simulink library "lightbar"  (Simulink 8.2)
settings: Solver=ode1  StartTime=0.0  StopTime=Inf  FixedStep=0.001  RelTol=1e-3
PostLoadFcn:
  | , if any(exist('dsrtsu_mdlpostloadfcn', 'file') == [2, 3, 6]), try dsrtsu_mdlpostloadfcn('Execute', bdroot); catch fprintf('Error in PostLoadFcn (dsrtsu_mdlpostloadfcn) for model "%s":\n %s\n', bdroot, lasterr); end, end,
libraries: lightbar x5, simulink x3, srx_platform x2, dsrc_transmitter x1
settings Model: DSRTSU_INTERNAL_RTI_VER=440  DSRTSU_INTERNAL_RTI_TYPE=rti1401  DSRTSU_INTERNAL_RTIFPGA=30  Creator=Admin  LastModifiedBy=Admin

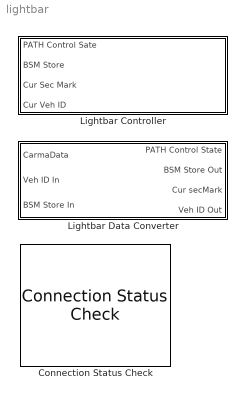
== system lightbar ==
  Connection Status Check : lightbar/Lightbar Controller/Light Control Logic/Connection Check/Connection Status Check
  Lightbar Controller : Subsystem
  Lightbar Data Converter : Subsystem

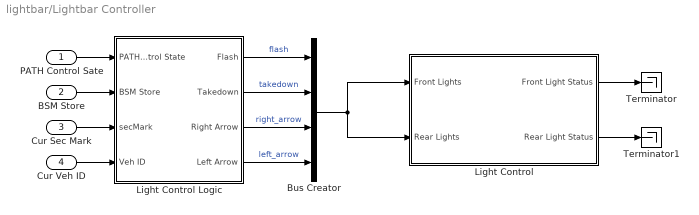
== system lightbar/Lightbar Controller ==
  PATH Control Sate : Inport
  BSM Store : Inport  Port=2
  Cur Sec Mark : Inport  Port=3
  Cur Veh ID : Inport  Port=4
  Bus Creator : BusCreator  Inputs='flash','takedown','right_arrow','left_arrow'  OutDataTypeStr=Bus: LightCommandBus  NonVirtualBus=on
  Light Control : Subsystem
  Light Control Logic : Subsystem
  Terminator : Terminator
  Terminator1 : Terminator
  wires:
  Bus Creator/1 -> Light Control/1(Front Lights), Light Control/2(Rear Lights)
  Light Control Logic/1(Flash) -> Bus Creator/1  "flash"
  Light Control Logic/2(Takedown) -> Bus Creator/2  "takedown"
  Light Control Logic/3(Right Arrow) -> Bus Creator/3  "right_arrow"
  Light Control Logic/4(Left Arrow) -> Bus Creator/4  "left_arrow"
  Light Control/1(Front Light Status) -> Terminator/1
  Light Control/2(Rear Light Status) -> Terminator1/1
  PATH Control Sate/1 -> Light Control Logic/1(PATH Control State)
  BSM Store/1 -> Light Control Logic/2(BSM Store)
  Cur Sec Mark/1 -> Light Control Logic/3(secMark)
  Cur Veh ID/1 -> Light Control Logic/4(Veh ID)

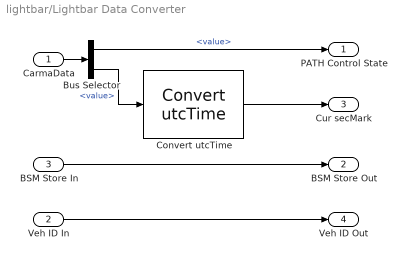
== system lightbar/Lightbar Data Converter ==
  CarmaData : Inport  OutDataTypeStr=Bus: GlobalStoreBus
  Veh ID In : Inport  Port=2
  BSM Store In : Inport  Port=3
  Bus Selector : BusSelector  OutputSignals=path_ctrl_status.value,global_utc_time_s.value
  Convert utcTime : dsrc_transmitter/BSM Broadcast/Convert TORC Data/Data Conversion/Convert utcTime
  PATH Control State : Outport
  BSM Store Out : Outport  Port=2
  Cur secMark : Outport  Port=3
  Veh ID Out : Outport  Port=4
  wires:
  CarmaData/1 -> Bus Selector/1
  Bus Selector/1 -> PATH Control State/1  "<value>"
  Veh ID In/1 -> Veh ID Out/1
  Convert utcTime/1 -> Cur secMark/1
  Bus Selector/2 -> Convert utcTime/1  "<value>"
  BSM Store In/1 -> BSM Store Out/1

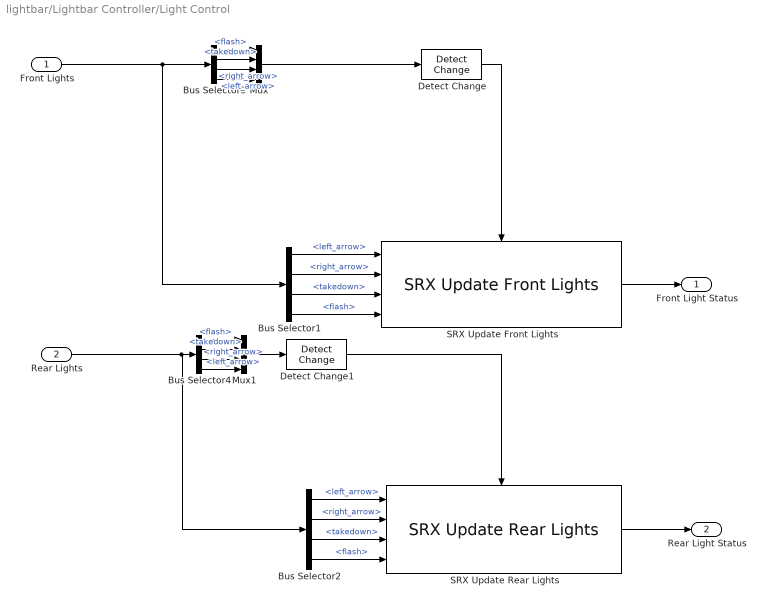
== system lightbar/Lightbar Controller/Light Control ==
  Front Lights : Inport  OutDataTypeStr=Bus: LightCommandBus
  Rear Lights : Inport  Port=2  OutDataTypeStr=Bus: LightCommandBus
  Bus Selector1 : BusSelector  OutputSignals=left_arrow,right_arrow,takedown,flash
  Bus Selector2 : BusSelector  OutputSignals=left_arrow,right_arrow,takedown,flash
  Bus Selector3 : BusSelector  OutputSignals=flash,takedown,right_arrow,left_arrow
  Bus Selector4 : BusSelector  OutputSignals=flash,takedown,right_arrow,left_arrow
  Detect Change : simulink/Logic and Bit Operations/Detect Change  vinit=0  InputProcessing=Inherited  OutDataTypeStr=boolean
  Detect Change1 : simulink/Logic and Bit Operations/Detect Change  vinit=0  InputProcessing=Inherited  OutDataTypeStr=boolean
  Mux : Mux
  Mux1 : Mux
  SRX Update Front Lights : srx_platform/SRX Update Front Lights
  SRX Update Rear Lights : srx_platform/SRX Update Rear Lights
  Front Light Status : Outport
  Rear Light Status : Outport  Port=2
  wires:
  Bus Selector4/4 -> Mux1/4  "<left_arrow>"
  Mux1/1 -> Detect Change1/1
  Bus Selector4/1 -> Mux1/1  "<flash>"
  Bus Selector4/2 -> Mux1/2  "<takedown>"
  Bus Selector4/3 -> Mux1/3  "<right_arrow>"
  Bus Selector3/2 -> Mux/2  "<takedown>"
  Bus Selector3/3 -> Mux/3  "<right_arrow>"
  Bus Selector3/4 -> Mux/4  "<left_arrow>"
  Mux/1 -> Detect Change/1
  SRX Update Rear Lights/1 -> Rear Light Status/1
  SRX Update Front Lights/1 -> Front Light Status/1
  Detect Change1/1 -> SRX Update Rear Lights/Enable
  Bus Selector2/1 -> SRX Update Rear Lights/1  "<left_arrow>"
  Bus Selector2/2 -> SRX Update Rear Lights/2  "<right_arrow>"
  Bus Selector2/3 -> SRX Update Rear Lights/3  "<takedown>"
  Rear Lights/1 -> Bus Selector4/1, Bus Selector2/1
  Bus Selector1/2 -> SRX Update Front Lights/2  "<right_arrow>"
  Bus Selector1/4 -> SRX Update Front Lights/4  "<flash>"
  Bus Selector1/3 -> SRX Update Front Lights/3  "<takedown>"
  Bus Selector1/1 -> SRX Update Front Lights/1  "<left_arrow>"
  Detect Change/1 -> SRX Update Front Lights/Enable
  Front Lights/1 -> Bus Selector1/1, Bus Selector3/1
  Bus Selector3/1 -> Mux/1  "<flash>"
  Bus Selector2/4 -> SRX Update Rear Lights/4  "<flash>"

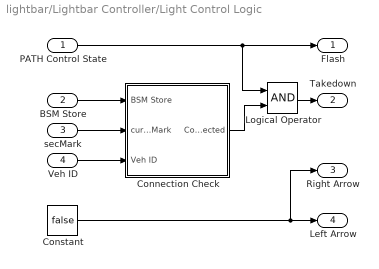
== system lightbar/Lightbar Controller/Light Control Logic ==
  PATH Control State : Inport
  BSM Store : Inport  Port=2
  secMark : Inport  Port=3
  Veh ID : Inport  Port=4
  Connection Check : Subsystem
  Constant : Constant  Value=false
  Logical Operator : Logic  AllPortsSameDT=off  OutDataTypeStr=boolean
  Flash : Outport
  Takedown : Outport  Port=2
  Right Arrow : Outport  Port=3
  Left Arrow : Outport  Port=4
  wires:
  PATH Control State/1 -> Logical Operator/1, Flash/1
  BSM Store/1 -> Connection Check/1(BSM Store)
  Connection Check/1(Connected) -> Logical Operator/2
  Constant/1 -> Right Arrow/1, Left Arrow/1
  Veh ID/1 -> Connection Check/3(Veh ID)
  Logical Operator/1 -> Takedown/1
  secMark/1 -> Connection Check/2(curSecMark)

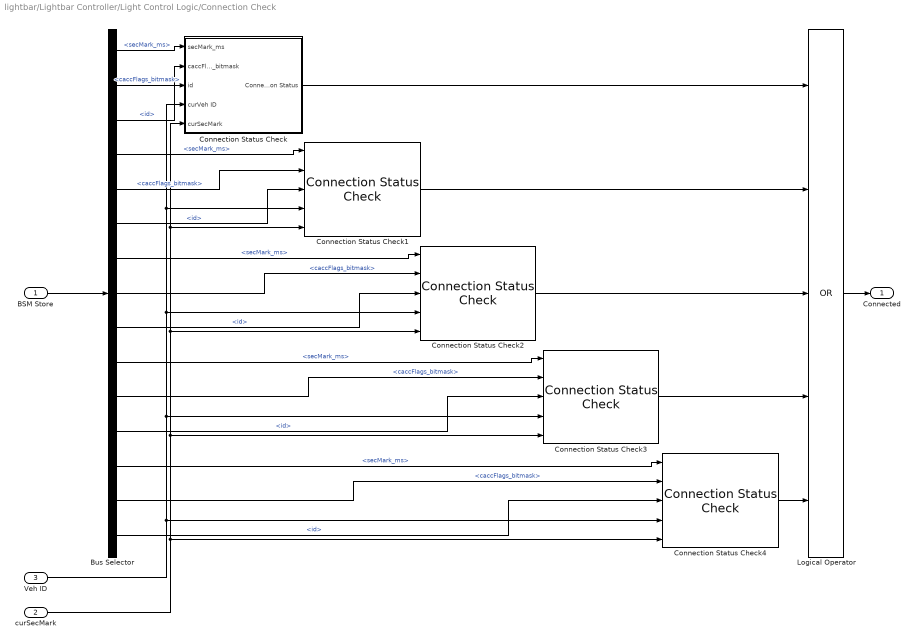
== system lightbar/Lightbar Controller/Light Control Logic/Connection Check ==
  BSM Store : Inport
  curSecMark : Inport  Port=2
  Veh ID : Inport  Port=3
  Bus Selector : BusSelector  OutputSignals=Veh5BSM.secMark_ms,Veh5BSM.caccFlags_bitmask,Veh5BSM.id,Veh4BSM.secMark_ms,Veh4BSM.caccFlags_bitmask,Veh4BSM.id,Veh3BSM.secMark_ms,Veh3BSM.caccFlags_bitmask,Veh3BSM.id,Veh2BSM.secMark_ms,Veh2BSM.caccFlags_bitmask,Veh2BSM.id,Veh1BSM.secMark_ms,Veh1BSM.caccFlags_bitmask,Veh1BSM.id
  Connection Status Check : Subsystem
  Connection Status Check{1..4} (4 alike) : lightbar/Lightbar Controller/Light Control Logic/Connection Check/Connection Status Check
  Logical Operator : Logic  Operator=OR  Inputs=5  AllPortsSameDT=off  OutDataTypeStr=boolean
  Connected : Outport
  wires:
  BSM Store/1 -> Bus Selector/1
  Bus Selector/1 -> Connection Status Check/1(secMark_ms)  "<secMark_ms>"
  Bus Selector/2 -> Connection Status Check/2(caccFlags_bitmask)  "<caccFlags_bitmask>"
  Bus Selector/3 -> Connection Status Check/3(id)  "<id>"
  Veh ID/1 -> Connection Status Check4/4, Connection Status Check3/4, Connection Status Check2/4, Connection Status Check1/4, Connection Status Check/4(curVeh ID)
  Logical Operator/1 -> Connected/1
  Connection Status Check/1("Connection Status ") -> Logical Operator/1
  curSecMark/1 -> Connection Status Check4/5, Connection Status Check3/5, Connection Status Check2/5, Connection Status Check1/5, Connection Status Check/5(curSecMark)
  Connection Status Check4/1 -> Logical Operator/5
  Connection Status Check3/1 -> Logical Operator/4
  Connection Status Check2/1 -> Logical Operator/3
  Connection Status Check1/1 -> Logical Operator/2
  Bus Selector/4 -> Connection Status Check1/1  "<secMark_ms>"
  Bus Selector/5 -> Connection Status Check1/2  "<caccFlags_bitmask>"
  Bus Selector/6 -> Connection Status Check1/3  "<id>"
  Bus Selector/7 -> Connection Status Check2/1  "<secMark_ms>"
  Bus Selector/8 -> Connection Status Check2/2  "<caccFlags_bitmask>"
  Bus Selector/9 -> Connection Status Check2/3  "<id>"
  Bus Selector/10 -> Connection Status Check3/1  "<secMark_ms>"
  Bus Selector/11 -> Connection Status Check3/2  "<caccFlags_bitmask>"
  Bus Selector/12 -> Connection Status Check3/3  "<id>"
  Bus Selector/13 -> Connection Status Check4/1  "<secMark_ms>"
  Bus Selector/14 -> Connection Status Check4/2  "<caccFlags_bitmask>"
  Bus Selector/15 -> Connection Status Check4/3  "<id>"

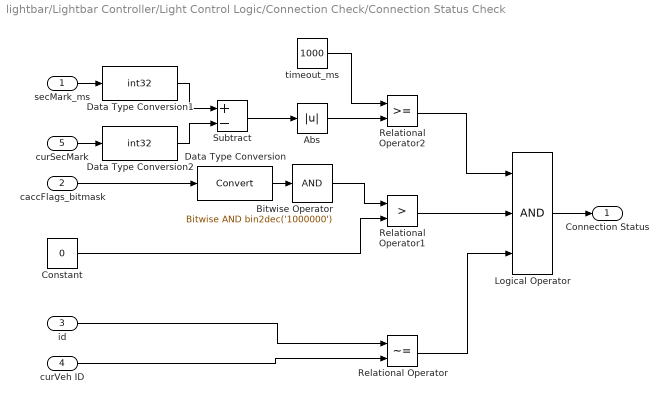
== system lightbar/Lightbar Controller/Light Control Logic/Connection Check/Connection Status Check ==
  secMark_ms : Inport
  caccFlags_bitmask : Inport  Port=2
  id : Inport  Port=3
  curVeh ID : Inport  Port=4
  curSecMark : Inport  Port=5
  Abs : Abs
  Bitwise Operator : simulink/Logic and Bit Operations/Bitwise Operator  logicop=AND  UseBitMask=on  BitMask=bin2dec('1000000')  BitMaskRealWorld=Stored Integer
  Constant : Constant  Value=0  OutDataTypeStr=uint32
  Data Type Conversion : DataTypeConversion
  Data Type Conversion1 : DataTypeConversion  OutDataTypeStr=int32
  Data Type Conversion2 : DataTypeConversion  OutDataTypeStr=int32
  Logical Operator : Logic  Inputs=3  AllPortsSameDT=off  OutDataTypeStr=boolean
  Relational Operator : RelationalOperator  Operator=~=  OutDataTypeStr=boolean
  Relational Operator1 : RelationalOperator  Operator=>  OutDataTypeStr=boolean
  Relational Operator2 : RelationalOperator  OutDataTypeStr=boolean
  Subtract : Sum  Inputs=+-  OutDataTypeStr=int32
  timeout_ms : Constant  Value=1000  OutDataTypeStr=uint32
  "Connection Status " : Outport
  wires:
  id/1 -> Relational Operator/1
  curVeh ID/1 -> Relational Operator/2
  Relational Operator/1 -> Logical Operator/3
  caccFlags_bitmask/1 -> Data Type Conversion/1
  Bitwise Operator/1 -> Relational Operator1/1
  Constant/1 -> Relational Operator1/2
  Relational Operator1/1 -> Logical Operator/2
  Data Type Conversion/1 -> Bitwise Operator/1
  Logical Operator/1 -> "Connection Status "/1
  secMark_ms/1 -> Data Type Conversion1/1
  curSecMark/1 -> Data Type Conversion2/1
  Subtract/1 -> Abs/1
  Abs/1 -> Relational Operator2/2
  timeout_ms/1 -> Relational Operator2/1
  Relational Operator2/1 -> Logical Operator/1
  Data Type Conversion1/1 -> Subtract/1
  Data Type Conversion2/1 -> Subtract/2
